simulink model "Mdl_Tacho"  (R2024b)
settings: Solver=FixedStepDiscrete  StartTime=0.0  StopTime=10.0  FixedStep=0.1  RelTol=1e-3  EnableMultiTasking=on
values from neighbouring files (symbols this model uses):
  EQUIPPED_FLAG = mpt.Parameter    [Mdl_Tacho_DD.m]
  HV_NE = mpt.Parameter    [Mdl_Tacho_DD.m]
  MCUID0025 = mpt.Parameter    [Mdl_Tacho_DD.m]
  MCUID0025_MAX = mpt.Parameter    [Mdl_Tacho_DD.m]
  MCUID0639 = mpt.Parameter    [Mdl_Tacho_DD.m]
  MCUID0640 = mpt.Parameter    [Mdl_Tacho_DD.m]
  Mdl_Tacho_cTaskPeriod = mpt.Parameter    [Mdl_Tacho_rte_types.m]
  N1 = mpt.Parameter    [Mdl_Tacho_DD.m]
  N2 = mpt.Parameter    [Mdl_Tacho_DD.m]
  NE1 = mpt.Parameter    [Mdl_Tacho_DD.m]
  NE_MET = mpt.Parameter    [Mdl_Tacho_DD.m]
  NE_MET_INVALID = mpt.Parameter    [Mdl_Tacho_DD.m]
  PTSYS_48V = mpt.Parameter    [Mdl_Tacho_DD.m]
  PTSYS_CONV = mpt.Parameter    [Mdl_Tacho_DD.m]
  PTSYS_DEFAULT = mpt.Parameter    [Mdl_Tacho_DD.m]
  PTSYS_HV = mpt.Parameter    [Mdl_Tacho_DD.m]
  PTSYS_MOTORHV = mpt.Parameter    [Mdl_Tacho_DD.m]
  PTSYS_PHV = mpt.Parameter    [Mdl_Tacho_DD.m]
  PTSYS_S_S = mpt.Parameter    [Mdl_Tacho_DD.m]
  REDZONE_MAX_VAL = mpt.Parameter    [Mdl_Tacho_DD.m]
  REDZONE_MIN_VAL = mpt.Parameter    [Mdl_Tacho_DD.m]
  RTE_E_MAX_AGE_EXCEEDED = mpt.Parameter    [Mdl_Tacho_rte_types.m]
  RTE_E_NEVER_RECEIVED = mpt.Parameter    [Mdl_Tacho_rte_types.m]
  RTE_E_OK = mpt.Parameter    [Mdl_Tacho_rte_types.m]
  RZ_INIT_VAL = mpt.Parameter    [Mdl_Tacho_DD.m]
  SPD_THRESHOLD = mpt.Parameter    [Mdl_Tacho_DD.m]
  TACHO_070D = mpt.Parameter    [Mdl_Tacho_DD.m]
  TACHO_COUNT_INIT = mpt.Parameter    [Mdl_Tacho_DD.m]
  TACHO_COUNT_INIT_U16 = mpt.Parameter    [Mdl_Tacho_DD.m]
  TACHO_COUNT_ONE = mpt.Parameter    [Mdl_Tacho_DD.m]
  TACHO_COUNT_TWO = mpt.Parameter    [Mdl_Tacho_DD.m]
  TACHO_DEBOUNCE_TIME = mpt.Parameter    [Mdl_Tacho_DD.m]
  TACHO_DISABLE = mpt.Parameter    [Mdl_Tacho_DD.m]
  TACHO_ENABLE = mpt.Parameter    [Mdl_Tacho_DD.m]
  TACHO_F = mpt.Parameter    [Mdl_Tacho_DD.m]
  TACHO_FSPORT = mpt.Parameter    [Mdl_Tacho_DD.m]
  TACHO_GR = mpt.Parameter    [Mdl_Tacho_DD.m]
  TACHO_GRMN = mpt.Parameter    [Mdl_Tacho_DD.m]
  TACHO_HYS_MAX = mpt.Parameter    [Mdl_Tacho_DD.m]
  TACHO_HYS_MIN = mpt.Parameter    [Mdl_Tacho_DD.m]
  TACHO_OFF = mpt.Parameter    [Mdl_Tacho_DD.m]
  TACHO_ON = mpt.Parameter    [Mdl_Tacho_DD.m]
  TACHO_RES_DIVIDER = mpt.Parameter    [Mdl_Tacho_DD.m]
  TACHO_RESOLUTION = mpt.Parameter    [Mdl_Tacho_DD.m]
  TACHO_REV_PEAK_TIMER_ELAPSED = mpt.Parameter    [Mdl_Tacho_DD.m]
  TACHO_RPM_THRESHOLD = mpt.Parameter    [Mdl_Tacho_DD.m]
  TACHO_TEN = mpt.Parameter    [Mdl_Tacho_DD.m]
  TACHO_THRESHOLD = mpt.Parameter    [Mdl_Tacho_DD.m]
  TACHO_VAL_ONE = mpt.Parameter    [Mdl_Tacho_DD.m]
  TACHO_VAL_ONE_U16 = mpt.Parameter    [Mdl_Tacho_DD.m]
  TACHO_VAL_TEN = mpt.Parameter    [Mdl_Tacho_DD.m]
  TACHO_VAL_THREE = mpt.Parameter    [Mdl_Tacho_DD.m]
  TACHO_VAL_TWENTY = mpt.Parameter    [Mdl_Tacho_DD.m]
  TACHO_VAL_ZERO = mpt.Parameter    [Mdl_Tacho_DD.m]
  TACHO_VAL_ZERO_U16 = mpt.Parameter    [Mdl_Tacho_DD.m]
  TACHO_VAL_ZERO_U32 = mpt.Parameter    [Mdl_Tacho_DD.m]
  VAL_ONE = mpt.Parameter    [Mdl_Tacho_DD.m]
  VAL_ZERO = mpt.Parameter    [Mdl_Tacho_DD.m]
undefined symbols (not defined in the file or in its folder): CLUSTER_ACTIVE, CLUSTER_INACTIVE, eEngineSpeedIn, eFUNC_NORTH_AMERICA, eJust_Received, eSIGNAL_MISSING, eSIGNAL_NEVER_RECEIVED, IgnOff, IgnOn, NE1_Recieve_Notify_Value, NE1_SignalVal, pJustRcvdStatus, RxCan_SignalClearJustRcvdStatus, RxCan_SignalGetJustRcvdStatus, RxCan_SignalInvalidProcessingControl, RxCan_SignalMissingProcessingControl, RxCan_SignalNRProcessingControl, SignalId, Status, tRxSignalId_type_instance, tRxSignalJustRcvdStatus_type_instance, tRxSignalStatus_type_instance
libraries: simulink x23
(part 3 of 3)

== system Mdl_Tacho/Mdl_Tacho_Task_sys/Subsystem/If Action Subsystem/Subsystem/Subsystem1/If Action Subsystem ==
  Action Port : ActionPort  ActionPortLabel=if(u1 < u2)
  Add : Sum
  Constant : Constant  Value=TACHO_COUNT_ONE
  Data Store Read : DataStoreRead  DataStoreName=DigitalTacho__Out  IndexOptions=Index vector (dialog)  Indices=1  OutputSizes=1
  Data Store Read1 : DataStoreRead  DataStoreName=DigtalTachoBuffIndex  IndexOptions=Index vector (dialog)  Indices=1  OutputSizes=1
  Data Store Write : DataStoreWrite  DataStoreName=DigtalTachoBuffIndex  IndexOptions=Index vector (dialog)  Indices=1  OutputSizes=1
  Digital_Tacho_Out : Outport  VectorParamsAs1DForOutWhenUnconnected=off
  wires:
  Constant/1 -> Add/2
  Add/1 -> Data Store Write/1
  Data Store Read1/1 -> Add/1
  Data Store Read/1 -> Digital_Tacho_Out/1

== system Mdl_Tacho/Mdl_Tacho_Task_sys/Subsystem/If Action Subsystem/Subsystem/Subsystem1/If Action Subsystem1 ==
  NE_IN_ForDigitalTacho_In : Inport
  Action Port : ActionPort  ActionPortLabel=else
  Constant : Constant  Value=TACHO_COUNT_INIT
  Constant9 : Constant  Value=TACHO_VAL_ZERO_U32  LockScale=on
  Data Store Write : DataStoreWrite  DataStoreName=DigtalTachoBuffIndex  IndexOptions=Index vector (dialog)  Indices=1  OutputSizes=1
  Data Store Write4 : DataStoreWrite  DataStoreName=fl_digital_odo_Sum  IndexOptions=Index vector (dialog)  Indices=1  OutputSizes=1
  For Iterator Subsystem : Subsystem  TreatAsAtomicUnit=on
  NE_IN_ForDigitalTacho__Out : Outport  VectorParamsAs1DForOutWhenUnconnected=off
  wires:
  Constant/1 -> Data Store Write/1
  NE_IN_ForDigitalTacho_In/1 -> For Iterator Subsystem/1(NE_IN_ForDigitalTacho_In)
  For Iterator Subsystem/1(NE_IN_ForDigitalTacho__Out) -> NE_IN_ForDigitalTacho__Out/1
  Constant9/1 -> Data Store Write4/1

== system Mdl_Tacho/Mdl_Tacho_Task_sys/Subsystem/If Action Subsystem/Average_Calculation/Subsystem/If Action Subsystem1/If Action Subsystem ==
  In1 : Inport
  Action Port : ActionPort  ActionPortLabel=if(u1 ~= 0)
  Add : Sum  OutDataTypeStr=uint16  AccumDataTypeStr=uint16  RndMeth=Simplest
  Constant2 : Constant  Value=TACHO_HYS_MIN
  Out1 : Outport  VectorParamsAs1DForOutWhenUnconnected=off
  wires:
  Add/1 -> Out1/1
  In1/1 -> Add/1
  Constant2/1 -> Add/2

== system Mdl_Tacho/Mdl_Tacho_Task_sys/Subsystem/If Action Subsystem/Average_Calculation/Subsystem/If Action Subsystem1/If Action Subsystem1 ==
  Current_NE_AVG1 : Inport
  Action Port : ActionPort  ActionPortLabel=elseif(u2 ~= 0)
  Constant2 : Constant  Value=TACHO_HYS_MIN
  Subtract : Sum  Inputs=+-  OutDataTypeStr=uint16  AccumDataTypeStr=uint16  RndMeth=Simplest
  Out2 : Outport  VectorParamsAs1DForOutWhenUnconnected=off
  wires:
  Current_NE_AVG1/1 -> Subtract/1
  Subtract/1 -> Out2/1
  Constant2/1 -> Subtract/2

== system Mdl_Tacho/Mdl_Tacho_Task_sys/Subsystem/If Action Subsystem/Average_Calculation/Subsystem/If Action Subsystem1/If Action Subsystem2 ==
  Old_NE_Avg : Inport
  Action Port : ActionPort  ActionPortLabel=else
  Out1 : Outport  VectorParamsAs1DForOutWhenUnconnected=off
  wires:
  Old_NE_Avg/1 -> Out1/1

== system Mdl_Tacho/Mdl_Tacho_Task_sys/Subsystem/If Action Subsystem/Subsystem/Subsystem1/If Action Subsystem1/For Iterator Subsystem ==
  NE_IN_ForDigitalTacho_In : Inport
  Constant : Constant  Value=TACHO_VAL_THREE
  Data Store Read : DataStoreRead  DataStoreName=fl_digital_odo_Sum  IndexOptions=Index vector (dialog)  Indices=1  OutputSizes=1
  Data Store Write4 : DataStoreWrite  DataStoreName=fl_digital_odo_Sum  IndexOptions=Index vector (dialog)  Indices=1  OutputSizes=1
  Divide : Product  Inputs=*/  OutDataTypeStr=uint16  SaturateOnIntegerOverflow=on
  For Iterator : ForIterator  ResetStates=reset  IterationLimit=TACHO_COUNT_THREE_INT  IndexMode=Zero-based  IterationVariableDataType=int8
  Selector : Selector  IndexMode=Zero-based  InputPortWidth=3  IndexOptions=Index vector (port)  Indices=[1 3]  OutputSizes=1
  Sum : Sum  Inputs=|++  SaturateOnIntegerOverflow=on
  NE_IN_ForDigitalTacho__Out : Outport  VectorParamsAs1DForOutWhenUnconnected=off
  wires:
  For Iterator/1 -> Selector/2
  NE_IN_ForDigitalTacho_In/1 -> Selector/1
  Selector/1 -> Sum/1
  Sum/1 -> Divide/1, Data Store Write4/1
  Data Store Read/1 -> Sum/2
  Constant/1 -> Divide/2
  Divide/1 -> NE_IN_ForDigitalTacho__Out/1

== matlab function Mdl_Tacho/Mdl_Tacho_Task_sys/Subsystem/If Action Subsystem/Enabled Subsystem/Rev peak end check/Rev peak end check ==
  data: NE_AVE2 input; RevPeakOnOff data_store_memory; RevPeakValue data_store_memory; TACHO_ON parameter; TACHO_OFF parameter; RevPeak_timer data_store_memory; RevPeakTimer_Plus_One input; TACHO_REV_PEAK_TIMER_ELAPSED parameter
function fcn(NE_AVE2, TACHO_ON, TACHO_OFF, RevPeakTimer_Plus_One, TACHO_REV_PEAK_TIMER_ELAPSED)

aVarTruthTableCondition_1 = false;
aVarTruthTableCondition_2 = false;


% RevPeakOnOff flag is off

aVarTruthTableCondition_1 = logical((RevPeakOnOff == TACHO_OFF));

% RevPeakOnOff is ON and NE_AVE2 > RevPeakValue

aVarTruthTableCondition_2 = logical(((NE_AVE2>RevPeakValue) || (RevPeak_timer >= TACHO_REV_PEAK_TIMER_ELAPSED)));

if (aVarTruthTableCondition_1)
    aFcnTruthTableAction_1();
elseif (aVarTruthTableCondition_2)
    aFcnTruthTableAction_2();
else % Default
    aFcnTruthTableAction_3();
end

function aFcnTruthTableAction_1()

% While RevPeakOnOff No Change

RevPeakValue = TACHO_OFF;
RevPeak_Timer = TACHO_OFF;
RevPeakOnOff = RevPeakOnOff;

function aFcnTruthTableAction_2()

% While RevPeakOnOff Off

RevPeakOnOff = TACHO_OFF;
RevPeakValue = TACHO_OFF;
RevPeak_Timer = TACHO_OFF;

function aFcnTruthTableAction_3()

% No Change

RevPeakOnOff = RevPeakOnOff;
RevPeakValue = RevPeakValue;
RevPeak_Timer = RevPeakTimer_Plus_One;

== matlab function Mdl_Tacho/Mdl_Tacho_Task_sys/Subsystem/If Action Subsystem/Accumulation_Processing/Truth Table1 ==
  data: New_NE_Input input; NE_MET_Value input; HV_NE_Value input; HV_NE_Status input; NE1_Status input; NE1_Value input; NE_MET_Status input; RTE_E_MAX_AGE_EXCEEDED parameter; RTE_E_NEVER_RECEIVED parameter; RTE_E_OK parameter; NE1 parameter; HV_NE parameter; NE_MET parameter; NE_In output uint16; NE1_COMStatus input; NE_MET_INVALID parameter
function NE_In = fcn(New_NE_Input, NE_MET_Value, HV_NE_Value, HV_NE_Status, NE1_Status, NE1_Value, NE_MET_Status, RTE_E_MAX_AGE_EXCEEDED, RTE_E_NEVER_RECEIVED, RTE_E_OK, NE1, HV_NE, NE_MET, NE1_COMStatus, NE_MET_INVALID)

aVarTruthTableCondition_1 = false;
aVarTruthTableCondition_2 = false;
aVarTruthTableCondition_3 = false;
aVarTruthTableCondition_4 = false;
aVarTruthTableCondition_5 = false;
aVarTruthTableCondition_6 = false;
aVarTruthTableCondition_7 = false;
aVarTruthTableCondition_8 = false;
aVarTruthTableCondition_9 = false;


% NE_MET Invalid Condition

aVarTruthTableCondition_1 = logical(((New_NE_Input == NE_MET) && (NE_MET_Status == RTE_E_MAX_AGE_EXCEEDED) && ((NE1_Status == RTE_E_MAX_AGE_EXCEEDED) || (NE1_COMStatus == RTE_E_NEVER_RECEIVED))));

% NE1 valid condition in NE_MET variant

aVarTruthTableCondition_2 = logical(((New_NE_Input == NE_MET) && (NE_MET_Status == RTE_E_MAX_AGE_EXCEEDED) && (NE1_Status == RTE_E_OK)));

% NE_MET Invalid Condition

aVarTruthTableCondition_3 = logical(((New_NE_Input == NE_MET) && (NE_MET_Status == RTE_E_OK)  && (NE_MET_Value == NE_MET_INVALID) && ((NE1_Status == RTE_E_MAX_AGE_EXCEEDED) || (NE1_COMStatus == RTE_E_NEVER_RECEIVED))));

% NE1 valid condition in NE_MET variant

aVarTruthTableCondition_4 = logical(((New_NE_Input == NE_MET) && (NE_MET_Status == RTE_E_OK)  && (NE_MET_Value == NE_MET_INVALID) && (NE1_Status ==RTE_E_OK)));

% NE_MET Valid condition

aVarTruthTableCondition_5 = logical(((New_NE_Input == NE_MET) && (NE_MET_Status == RTE_E_OK)   && (NE_MET_Value ~= NE_MET_INVALID)));

% HV_NE invalid condition

aVarTruthTableCondition_6 = logical(((New_NE_Input == HV_NE) && (HV_NE_Status == RTE_E_MAX_AGE_EXCEEDED)   &&  ((NE1_Status == RTE_E_MAX_AGE_EXCEEDED) || (NE1_COMStatus == RTE_E_NEVER_RECEIVED))));

% NE1 valid condition in HV_NE variant

aVarTruthTableCondition_7 = logical(((New_NE_Input == HV_NE) && (HV_NE_Status == RTE_E_MAX_AGE_EXCEEDED)   &&  (NE1_Status == RTE_E_OK)));

% HV_NE valid condition

aVarTruthTableCondition_8 = logical(((New_NE_Input == HV_NE) && (HV_NE_Status == RTE_E_OK)));

% NE1 invalid condition

aVarTruthTableCondition_9 = logical(((New_NE_Input == NE1) && ((NE1_Status == RTE_E_MAX_AGE_EXCEEDED) || (NE1_COMStatus == RTE_E_NEVER_RECEIVED))));

if (aVarTruthTableCondition_1)
    aFcnTruthTableAction_1();
elseif (aVarTruthTableCondition_2)
    aFcnTruthTableAction_4();
elseif (aVarTruthTableCondition_3)
    aFcnTruthTableAction_1();
elseif (aVarTruthTableCondition_4)
    aFcnTruthTableAction_4();
elseif (aVarTruthTableCondition_5)
    aFcnTruthTableAction_3();
elseif (aVarTruthTableCondition_6)
    aFcnTruthTableAction_1();
elseif (aVarTruthTableCondition_7)
    aFcnTruthTableAction_4();
elseif (aVarTruthTableCondition_8)
    aFcnTruthTableAction_2();
elseif (aVarTruthTableCondition_9)
    aFcnTruthTableAction_1();
else % Default
    aFcnTruthTableAction_4();
end

function aFcnTruthTableAction_1()

% Tachometer failure Action

NE_In = 0;

function aFcnTruthTableAction_2()

% Tachometer HV_NE valid Action

NE_In = HV_NE_Value;

function aFcnTruthTableAction_3()

% Tachometer NE_MET valid Action

NE_In = NE_MET_Value;

function aFcnTruthTableAction_4()

% Tachometer NE1 valid Action

NE_In = NE1_Value;

== matlab function Mdl_Tacho/Mdl_Tacho_Task_sys/Subsystem/If Action Subsystem/Input_Determination/Truth Table ==
  data: NE_MET_Ex input; New_NE_Input output uint16; HV_NE_Ex input; NE1 parameter; NE_MET parameter; HV_NE parameter; EQUIPPED_FLAG parameter
function New_NE_Input = fcn(NE_MET_Ex, HV_NE_Ex, NE1, NE_MET, HV_NE, EQUIPPED_FLAG)

aVarTruthTableCondition_1 = false;
aVarTruthTableCondition_2 = false;


% Check NE_MET is configured

aVarTruthTableCondition_1 = logical((NE_MET_Ex == EQUIPPED_FLAG));

% Check HV_NE is configured

aVarTruthTableCondition_2 = logical((HV_NE_Ex == EQUIPPED_FLAG));

if (aVarTruthTableCondition_1)
    aFcnTruthTableAction_1();
elseif (aVarTruthTableCondition_2)
    aFcnTruthTableAction_2();
else % Default
    aFcnTruthTableAction_3();
end

function aFcnTruthTableAction_1()

% NE_MET Input Action

New_NE_Input = NE_MET;

function aFcnTruthTableAction_2()

% HV_NE Input Action

New_NE_Input = HV_NE;

function aFcnTruthTableAction_3()

% NE1 Input Action

New_NE_Input = NE1;

== matlab function Mdl_Tacho/Mdl_Tacho_Task_sys/Subsystem/Tachometer_applicable_flag ==
  data: PowerTrain_Flag input; Tachometer_applicable_flag output; PTSYS_CONV parameter; PTSYS_S_S parameter; PTSYS_HV parameter; PTSYS_PHV parameter; PTSYS_MOTORHV parameter; PTSYS_48V parameter; TACHO_ENABLE parameter; TACHO_DISABLE parameter; PTSYS_DEFAULT parameter
function Tachometer_applicable_flag = fcn(PowerTrain_Flag, PTSYS_CONV, PTSYS_S_S, PTSYS_HV, PTSYS_PHV, PTSYS_MOTORHV, PTSYS_48V, TACHO_ENABLE, TACHO_DISABLE, PTSYS_DEFAULT)

aVarTruthTableCondition_1 = false;


% Tacho gauge applicable check according to PTsys

aVarTruthTableCondition_1 = logical((PowerTrain_Flag == PTSYS_DEFAULT) || (PowerTrain_Flag == PTSYS_CONV) || (PowerTrain_Flag == PTSYS_S_S) || (PowerTrain_Flag == PTSYS_HV) || (PowerTrain_Flag == PTSYS_PHV) || (PowerTrain_Flag == PTSYS_MOTORHV)|| (PowerTrain_Flag == PTSYS_48V));

if (aVarTruthTableCondition_1)
    aFcnTruthTableAction_1();
else % Default
    aFcnTruthTableAction_2();
end

function aFcnTruthTableAction_1()

% Tacho applicable

Tachometer_applicable_flag = TACHO_ENABLE;

function aFcnTruthTableAction_2()

% Tacho not applicable

Tachometer_applicable_flag = TACHO_DISABLE;

== matlab function Mdl_Tacho/Mdl_Tacho_Task_sys/Subsystem/If Action Subsystem/RedZone Check ==
  data: B_RZRPM_Value input; RZ_ST output; B_RZRPM_Status input; fl_prev_RZ_ST_u8 input; REDZONE_MIN_VAL parameter; REDZONE_MAX_VAL parameter; RTE_E_MAX_AGE_EXCEEDED parameter; RTE_E_NEVER_RECEIVED parameter
function RZ_ST = fcn(B_RZRPM_Value, B_RZRPM_Status, fl_prev_RZ_ST_u8, REDZONE_MIN_VAL, REDZONE_MAX_VAL, RTE_E_MAX_AGE_EXCEEDED, RTE_E_NEVER_RECEIVED)

aVarTruthTableCondition_1 = false;
aVarTruthTableCondition_2 = false;
aVarTruthTableCondition_3 = false;


% Missing or Never received

aVarTruthTableCondition_1 = logical((B_RZRPM_Status == RTE_E_MAX_AGE_EXCEEDED) || ( B_RZRPM_Status == RTE_E_NEVER_RECEIVED));

% Red Zone Min Value Check

aVarTruthTableCondition_2 = logical(B_RZRPM_Value <= REDZONE_MIN_VAL);

% Red Zone Max Value Check

aVarTruthTableCondition_3 = logical(B_RZRPM_Value >= REDZONE_MAX_VAL);

if (aVarTruthTableCondition_1)
    aFcnTruthTableAction_1();
elseif (aVarTruthTableCondition_2)
    aFcnTruthTableAction_2();
elseif (aVarTruthTableCondition_3)
    aFcnTruthTableAction_3();
else % Default
    aFcnTruthTableAction_4();
end

function aFcnTruthTableAction_1()

% No Change

RZ_ST = fl_prev_RZ_ST_u8;

function aFcnTruthTableAction_2()

% Less than equal to Min Value

RZ_ST = REDZONE_MIN_VAL;

function aFcnTruthTableAction_3()

% Greater than equal to MAX Value

RZ_ST = REDZONE_MAX_VAL;

function aFcnTruthTableAction_4()

% Other than above inputs

RZ_ST = B_RZRPM_Value;

== matlab function Mdl_Tacho/Mdl_Tacho_Task_sys/Subsystem/If Action Subsystem/Truth HMI_TC_NEEDLE_TRANSPARENT ==
  data: HMI_TC_NEEDLE_TRANSPARENT output; NEMETFD_Value input; NEMETFD_Status input; RTE_E_MAX_AGE_EXCEEDED parameter; RTE_E_NEVER_RECEIVED parameter; TACHO_VAL_TEN parameter; TACHO_VAL_ZERO parameter
function HMI_TC_NEEDLE_TRANSPARENT = fcn(NEMETFD_Value, NEMETFD_Status, RTE_E_MAX_AGE_EXCEEDED, RTE_E_NEVER_RECEIVED, TACHO_VAL_TEN, TACHO_VAL_ZERO)

aVarTruthTableCondition_1 = false;


% Missing, Never recived and More than 10 Check

aVarTruthTableCondition_1 = logical((NEMETFD_Status == RTE_E_NEVER_RECEIVED) || (NEMETFD_Status == RTE_E_MAX_AGE_EXCEEDED )|| (NEMETFD_Value > TACHO_VAL_TEN));

if (aVarTruthTableCondition_1)
    aFcnTruthTableAction_1();
else % Default
    aFcnTruthTableAction_2();
end

function aFcnTruthTableAction_1()

% NEEDLE_TRANSPARENT Opaque

HMI_TC_NEEDLE_TRANSPARENT =  TACHO_VAL_ZERO;

function aFcnTruthTableAction_2()

% NEEDLE_TRANSPARENT Not Opaque

HMI_TC_NEEDLE_TRANSPARENT =  NEMETFD_Value;

== matlab function Mdl_Tacho/Mdl_Tacho_Task_sys/Subsystem/If Action Subsystem/Truth Table ==
  data: NVM_MCUID0025 input; Rev_peak_process_Status output; TACHO_GR parameter; TACHO_GRMN parameter; TACHO_FSPORT parameter; TACHO_F parameter; TACHO_070D parameter; TACHO_VAL_ZERO parameter; TACHO_VAL_ONE parameter
function Rev_peak_process_Status = fcn(NVM_MCUID0025, TACHO_GR, TACHO_GRMN, TACHO_FSPORT, TACHO_F, TACHO_070D, TACHO_VAL_ZERO, TACHO_VAL_ONE)

aVarTruthTableCondition_1 = false;


% Condition Check

aVarTruthTableCondition_1 = logical((NVM_MCUID0025 == TACHO_GR) || (NVM_MCUID0025 == TACHO_GRMN) || (NVM_MCUID0025 == TACHO_FSPORT) || (NVM_MCUID0025 == TACHO_F) || (NVM_MCUID0025 == TACHO_070D));

if (aVarTruthTableCondition_1)
    aFcnTruthTableAction_1();
else % Default
    aFcnTruthTableAction_2();
end

function aFcnTruthTableAction_1()

% Rev peak process Enable

Rev_peak_process_Status = TACHO_VAL_ONE;

function aFcnTruthTableAction_2()

% Rev peak process Disable

Rev_peak_process_Status = TACHO_VAL_ZERO;
